simulink model "MMSAR_SequentialNoZOH"  (R2021a)
settings: Solver=VariableStepAuto  StartTime=0.0  StopTime=40  RelTol=1e-3
values from neighbouring files (symbols this model uses):
  ADC_input = database_load('EEGdata_ch1.mat', epoch)    [Copy_of_MMSeqNoZOH_main.m]    (also in MMSeqNoZOH_main.m = database_load('EEGdata_ch1.mat',1)'/10; database_load.m = (2/1000*(selected-min(selected))/(max(selected)-min(selected)
  C2 = C1*cap_ratio    [Copy_of_MMSeqNoZOH_main.m]    (also in MMSeqNoZOH_main.m)
  Cf = minimum_cap    [Copy_of_MMSeqNoZOH_main.m]
  Cf_unit_cap = 20    [MMSeqNoZOH_main.m]
  clk_freq = 2.1*input_BW    (= 268.8)    [Copy_of_MMSeqNoZOH_main.m]    (also in MMSeqNoZOH_main.m = 537.6)
  clk_period = 1/clk_freq    (= 0.00372023809524)    [Copy_of_MMSeqNoZOH_main.m]    (also in MMSeqNoZOH_main.m = 0.00186011904762)
  comparator_high_offset = 0.2*10e-4    (= 0.0002)    [Copy_of_MMSeqNoZOH_main.m]    (also in MMSeqNoZOH_main.m = 0.008)
  comparator_low_offset = -.1*10e-4    (= -0.0001)    [Copy_of_MMSeqNoZOH_main.m]    (also in MMSeqNoZOH_main.m = 0.008)
  comparator_noise_on = noise_on    (= 1)    [Copy_of_MMSeqNoZOH_main.m]    (also in MMSeqNoZOH_main.m)
  comparator_noise_rms = 1*k*T* 2/3 / minimum_cap    [Copy_of_MMSeqNoZOH_main.m]    (also in MMSeqNoZOH_main.m = 3.50242438407e-06)
  comparator_offset_on = noise_on    (= 1)    [Copy_of_MMSeqNoZOH_main.m]    (also in MMSeqNoZOH_main.m)
  DAC_cap = max([minimum_sampling_cap, minimum_technology_cap, minimum_match_cap_DAC])    [MMSeqNoZOH_main.m]
  k = 1.38064852e-23    [Copy_of_MMSeqNoZOH_main.m]    (also in MMSeqNoZOH_main.m)
  leak_current = leakage_on * 2 *10^(-15)    (= 2e-15)    [MMSeqNoZOH_main.m]
  LNA_bandwidth = 3*input_BW    (= 384)    [Copy_of_MMSeqNoZOH_main.m]    (also in MMSeqNoZOH_main.m = 768)
  LNA_gain = 100    [Copy_of_MMSeqNoZOH_main.m]    (also in MMSeqNoZOH_main.m = 1000)
  LNA_noise_on = noise_on    (= 1)    [Copy_of_MMSeqNoZOH_main.m]    (also in MMSeqNoZOH_main.m)
  LNA_noise_vector = [pd.random(nb_MAC,1);0]'    [Copy_of_MMSeqNoZOH_main.m]    (also in MMSeqNoZOH_main.m)
  LNA_SR = I_LNA/(nb_activations*minimum_cap)    [Copy_of_MMSeqNoZOH_main.m]    (also in MMSeqNoZOH_main.m = I_LNA/(nb_activations*MAC_cap))
  MM_attenuation_coeff = 1    [Copy_of_MMSeqNoZOH_main.m]    (also in MMSeqNoZOH_main.m)
  MM_incomplete_transfer_coeff = C1/(C1+C2)    [Copy_of_MMSeqNoZOH_main.m]    (also in MMSeqNoZOH_main.m)
  MM_sampling_noise = noise_on*((k*T * C1/(C1+C2)^2) + (k*T*(C1*C2/(C1+C2))/C2^2))    [Copy_of_MMSeqNoZOH_main.m]    (also in MMSeqNoZOH_main.m)
  nb_MAC = 384    [Copy_of_MMSeqNoZOH_main.m]    (also in MMSeqNoZOH_main.m; negateLeakage.m = size(sensing_matrix,2))
  number_of_bits = 6    [Copy_of_MMSeqNoZOH_main.m]    (also in MMSeqNoZOH_main.m)
  sample_time_jitter = 16e-12    (= 1.6e-11)    [Copy_of_MMSeqNoZOH_main.m]    (also in MMSeqNoZOH_main.m)
  sampling_gain = Cs/Cf    [Copy_of_MMSeqNoZOH_main.m]    (also in MMSeqNoZOH_main.m = Cs_unit_cap/Cf_unit_cap)
  sampling_jitter_on = noise_on    (= 1)    [Copy_of_MMSeqNoZOH_main.m]    (also in MMSeqNoZOH_main.m)
  sim_number = 1    [Copy_of_MMSeqNoZOH_main.m]    (also in MMSeqNoZOH_main.m = 10)
  switch_noise_on = noise_on    (= 1)    [Copy_of_MMSeqNoZOH_main.m]    (also in MMSeqNoZOH_main.m)
  switching_noise = k*T/Cf    [Copy_of_MMSeqNoZOH_main.m]    (also in MMSeqNoZOH_main.m = 2.03450520833e-06)
  T = 293    [Copy_of_MMSeqNoZOH_main.m]    (also in MMSeqNoZOH_main.m)
  Vref = 2    [Copy_of_MMSeqNoZOH_main.m]    (also in MMSeqNoZOH_main.m)
  ZOH_delta = 0*Vref/(2^number_of_bits)    (= 0)    [MMSeqNoZOH_main.m]
libraries: dspsrcs4 x8, simulink x8, dspsigops x4, simulink_extras x4, spsFirstOrderFilterLib x2, dspswit3 x2
(part 2 of 2)

== matlab function MMSAR_SequentialNoZOH/Sensing Channel 1/MAC unit/MATLAB Function ==
  data: MAC_in input; signal_in input; MAC_out output; MM_attenuation input; MAC_element_in input; leak_current input; clk_freq input; hold_cap input; sensed input
function MAC_out = fcn(MAC_in, signal_in, MM_attenuation, MAC_element_in, leak_current, clk_freq, hold_cap, sensed)

if (MAC_element_in == 0)
    MAC_out = MAC_in;
else 
    MAC_out = signal_in*MAC_element_in + MM_attenuation*MAC_in;
end
if sensed==0 % Only leak if not sensed yet (in real implementation, it would be digitized. In this model, digitization always happens after full amount of cycles)
    MAC_out = max(0,MAC_out - leak_current/(clk_freq*hold_cap));
end
% MAC_out = MAC_out - leak_current/(clk_freq*hold_cap);
end

== matlab function MMSAR_SequentialNoZOH/Sensing Channel 2/SAR/DAC/DAC ==
  data: input_code input size=number_of_bits; out output double size=1; number_of_bits input; Vref input
function out = fcn(input_code, number_of_bits, Vref)
out = Vref/(2^number_of_bits) * (bi2de(input_code.', 'left-msb'));
end

== matlab function MMSAR_SequentialNoZOH/Sensing Channel 2/SAR/SAR/SAR ==
  data: output_code_decimal output size=1; output_code output size=number_of_bits; output_cycle output size=1; input_code_decimal input; cycle_in input; comparator_in input; number_of_bits input; done output
function [output_code_decimal, output_code, output_cycle, done] = fcn(input_code_decimal, cycle_in, comparator_in, number_of_bits)

    input_code = de2bi(input_code_decimal, 'left-msb');
    output_code = [zeros(number_of_bits-size(input_code.',1),1); input_code.'];


    if (cycle_in == number_of_bits)
        done = 1;
        output_code(number_of_bits,1) = comparator_in;
        output_cycle = 0;

    elseif (cycle_in == 0)

        output_code = zeros(number_of_bits,1);
        output_code(1, 1) = 1;
        done=0;
        output_cycle = 1;

    else

        if (comparator_in == 0)
            output_code(cycle_in,1) = 0;
        end

        output_code(cycle_in+1,1)=1;
        output_cycle = cycle_in+1;
        done=0;
    end
    output_code_decimal_temp = bi2de(output_code.', 'left-msb');
    output_code_decimal = output_code_decimal_temp(1,1);
end
